simulink model "Test"  (R2018a)
settings: Solver=VariableStepAuto  StartTime=0.0  StopTime=10.0  RelTol=1e-3
settings Model: Creator=wangluo  LastModifiedBy=wangluo

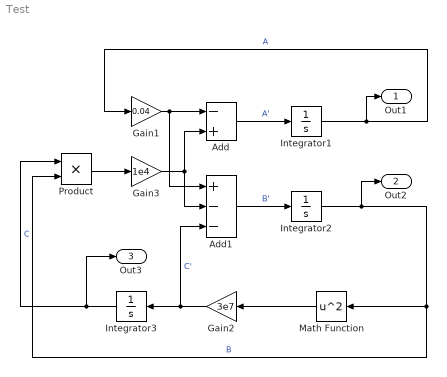
== system Test ==
  Add : Sum  Inputs=-+
  Add1 : Sum  Inputs=+--
  Gain1 : Gain  Gain=0.04
  Gain2 : Gain  Gain=3e7
  Gain3 : Gain  Gain=1e4
  Integrator1 : Integrator  InitialCondition=1
  Integrator2 : Integrator
  Integrator3 : Integrator
  Math Function : Math  Operator=square  SaturateOnIntegerOverflow=on
  Product : Product
  Out1 : Outport
  Out2 : Outport  Port=2
  Out3 : Outport  Port=3
  wires:
  Add1/1 -> Integrator2/1  "B'"
  Integrator2/1 -> Math Function/1, Product/2, Out2/1  "B"
  Add/1 -> Integrator1/1  "A'"
  Integrator1/1 -> Out1/1, Gain1/1  "A"
  Integrator3/1 -> Out3/1, Product/1  "C"
  Gain2/1 -> Add1/3, Integrator3/1  "C'"
  Math Function/1 -> Gain2/1
  Gain1/1 -> Add1/1, Add/1
  Gain3/1 -> Add1/2, Add/2
  Product/1 -> Gain3/1
